simulink model "crossroad"  (R2023a)
settings: Solver=VariableStepDiscrete  StartTime=21600  StopTime=54000  FixedStep=1  MinStep=1  RelTol=1e-3
InitFcn:
  | clear S_code; % Resetta variabili persistent di una funzione
  | clear controllore_code;
  | clear controllore_code_NN;
  | clear sensor_S12 sensor_S3;
libraries: truetime x5, fuzblock x2
settings Model: SimulationMode=accelerator  NumberOfSteps=5  Creator=simmt  LastModifiedBy=simmt

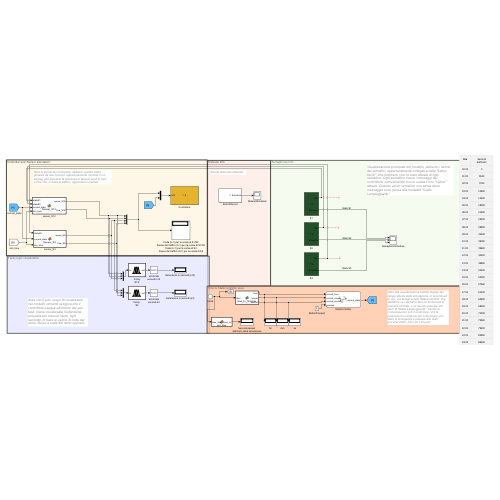
[thumbnail: Simulink's stored preview of the top-level diagram]
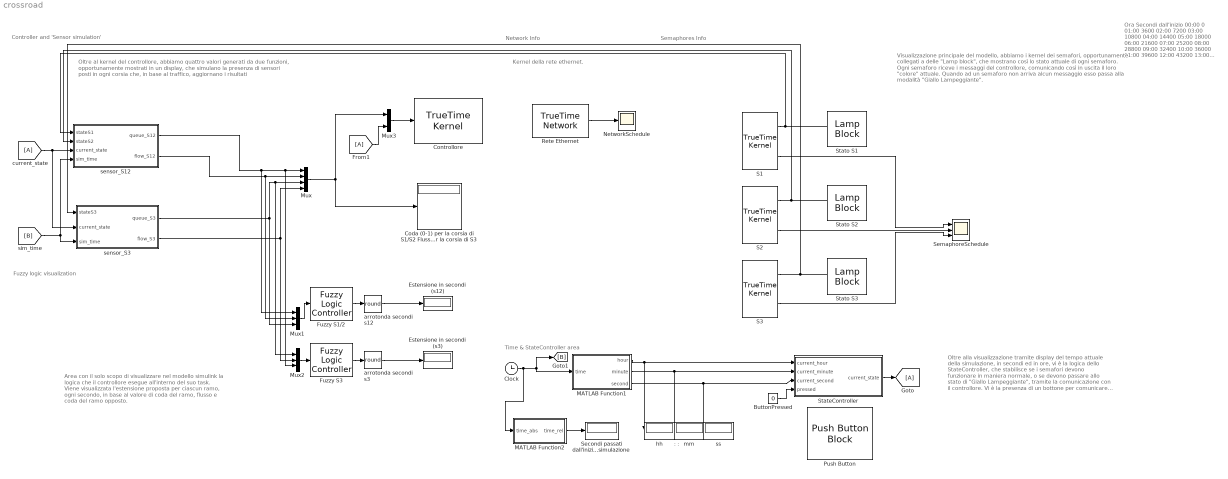
== system crossroad ==
  note: : :
  note: Ora
      | Secondi dall’inizio
      |
      | 00:00
      | 0
      |
      | 01:00
      | 3600
      |
      | 02:00
      | 7200
      |
      | 03:00
      | 10800
      |
      | 04:00
      | 14400
      |
      | 05:00
      | 18000
      |
      | 06:00
      | 21600
      |
      | 07:00
      | 25200
      |
      | 08:00
      | 28800
      |
      | 09:00
      | 32400
      |
      | 10:00
      | 36000
      |
      | 11:00
      | 39600
      |
      | 12:00
      | 43200
      |
      | 13:00
      | 46800
      |
      | 14:00
      | 50400
      |
      | 15:00
      | 54000
      |
      | 16:00
      | 57600
      |
      | 17:00
      | 61200
      |
      | 18:00
      | 64800
      |
      | 19:00
      | 68400
      |
      | 20:00
      | 72000
      |
      | 21:00
      | 75600
      |
      | 22:00
      | 79200
      |
      | 23:00
      | 82800
      |
      | 24:00
      | 86400
  note: Oltre al kernel del controllore, abbiamo quattro valori generati da due funzioni, opportunamente mostrati in un display, che simulano la presenza di sensori posti in ogni corsia che, in base al traffico, aggiornano i risultati
  note: Time & StateController area
  note: Controller and 'Sensor simulation'
  note: Semaphores Info
  note: Network Info
  note: Fuzzy logic visualization
  note: Area con il solo scopo di visualizzare nel modello simulink la logica che il controllore esegue all'interno del suo task. Viene visualizzata l'estensione proposta per ciascun ramo, ogni secondo, in base al valore di coda del ramo, flusso e coda del ramo opposto.
  note: Kernel della rete ethernet.
  note: Visualizzazione principale del modello, abbiamo i kernel dei semafori, opportunamente collegati a delle "Lamp block", che mostrano così lo stato attuale di ogni semaforo. Ogni semaforo riceve i messaggi del controllore, comunicando così in uscita il loro "colore" attuale. Quando ad un semaforo non arriva alcun messaggio esso passa alla modalità "Giallo Lampeggiante".
  note: Oltre alla visualizzazione tramite display del tempo attuale della simulazione, in secondi ed in ore, vi è la logica dello StateController, che stabilisce se i semafori devono funzionare in maniera normale, o se devono passare allo stato di "Giallo Lampeggiante", tramite la comunicazione con il controllore. Vi è la presenza di un bottone per comunicare uno stato di emergenza e passare allo stato poc'anzi citato. (clic con il mouse)
  "     mm     " : Display
  " ss" : Display
  ButtonPressed : Constant  Value=0  OutDataTypeStr=boolean
  Clock : Clock
  Coda (0-1) per la corsia di S1/S2 Flusso del traffico (0-1) per la corsia di S1/S2 Coda (0-1) per la corsia di S3 Flusso del traffico (0-1) per la corsia di S3 : Display
      settings: Format=bank
  Controllore : truetime/TrueTime Kernel  sfun=controllore_init  args=[]  ninputsoutputs=[5 0]  ntriggers=0  trigtype=falling  nwnodenbr=[1 4]  clockoffsetdrift=[0 0]  schedoutput=off  battery=off  poweroutput=off  label=1: 4
  Estensione in secondi (s12) : Display
      settings: Format=decimal (Stored Integer)
  Estensione in secondi (s3) : Display
  From1 : From
  Fuzzy S1/2 : fuzblock/Fuzzy Logic  Controller  FIS='green_extend.fis'  OutputSampleNumber=101  DataType=double  FuzzifiedInputs=off  RuleFiringStrengths=off  RuleOutputs=off  AggregatedOutputs=off  SimulateUsing=Interpreted execution  OutOfRangeInputValueMessage=warning  NoRuleFiredMessage=warning  EmptyOutputFuzzySetMessage=warning
  Fuzzy S3 : fuzblock/Fuzzy Logic  Controller  FIS='green_extend.fis'  OutputSampleNumber=101  DataType=double  FuzzifiedInputs=off  RuleFiringStrengths=off  RuleOutputs=off  AggregatedOutputs=off  SimulateUsing=Interpreted execution  OutOfRangeInputValueMessage=warning  NoRuleFiredMessage=warning  EmptyOutputFuzzySetMessage=warning
  Goto : Goto
  MATLAB Function1 : MATLAB Function  TreatAsAtomicUnit=on
  MATLAB Function2 : MATLAB Function  TreatAsAtomicUnit=on
  Mux : Mux
  Mux1 : Mux  Inputs=3
  Mux2 : Mux  Inputs=3
  Mux3 : Mux  Inputs=2
  NetworkSchedule : Scope
  Push Button : PushButtonBlock  ButtonText=Emergency  Icon=Hexagon  IconAlignment=Center  IconColor=On  OffValue=0.000000
  Rete Ethernet : truetime/TrueTime Network  nwtype=CSMA/CD (Ethernet)  nwnbr=1  nnodes=4  rate=20000000  minsize=512  lossprob=0.001  seed=42  bandwidths=[0.5 0.5]  slotsize=512  schedule=[1 1 2]  memsize=80000  buftype=Common buffer  overflow=Retransmit  dynSchedule=0  miniSlotSize=0  NIT=0  QSortMode=FIFO  sync=0  irtSchedule=0  nrtLength=0  nodeGraph=0  scheduleoutput=on
  S1 : truetime/TrueTime Kernel  sfun=S1_init  args=[]  ninputsoutputs=[0 1]  ntriggers=0  trigtype=falling  nwnodenbr=[1 1]  clockoffsetdrift=[0 0]  schedoutput=on  battery=off  poweroutput=off  label=1: 1
  S2 : truetime/TrueTime Kernel  sfun=S2_init  args=[]  ninputsoutputs=[0 1]  ntriggers=0  trigtype=falling  nwnodenbr=[1 2]  clockoffsetdrift=[0 0]  schedoutput=on  battery=off  poweroutput=off  label=1: 2
  S3 : truetime/TrueTime Kernel  sfun=S3_init  args=[]  ninputsoutputs=[0 1]  ntriggers=0  trigtype=falling  nwnodenbr=[1 3]  clockoffsetdrift=[0 0]  schedoutput=on  battery=off  poweroutput=off  label=1: 3
  Secondi passati dall'inizio della simulazione : Display
  SemaphoreSchedule : Scope  NumInputPorts=3
  StateController : Stateflow chart  TreatAsAtomicUnit=on
  Stato S1 : LampBlock  LabelPosition=Hide
  Stato S2 : LampBlock  LabelPosition=Hide
  Stato S3 : LampBlock  LabelPosition=Hide
  arrotonda secondi s12 : Rounding  Operator=round
  arrotonda secondi s3 : Rounding  Operator=round
  current_state : From
  hh : Display
  sensor_S12 : MATLAB Function  TreatAsAtomicUnit=on  SystemSampleTime=1
  sensor_S3 : MATLAB Function  TreatAsAtomicUnit=on  SystemSampleTime=1
  wires:
  sensor_S12/1(queue_S12) -> Mux1/1, Mux2/3, Mux/1
  Rete Ethernet/1 -> NetworkSchedule/1
  S3/2 -> SemaphoreSchedule/3
  S1/1 -> sensor_S12/1(stateS1)
  S2/1 -> sensor_S12/2(stateS2)
  S3/1 -> sensor_S3/1(stateS3)
  Mux/1 -> Coda (0-1) per la corsia di S1/S2 Flusso del traffico (0-1) per la corsia di S1/S2 Coda (0-1) per la corsia di S3 Flusso del traffico (0-1) per la corsia di S3/1, Mux3/1
  Clock/1 -> [B], MATLAB Function1/1(time), MATLAB Function2/1(time_abs)
  MATLAB Function1/1(hour) -> hh/1, StateController/1(current_hour)
  StateController/1(current_state) -> Goto/1
  S1/2 -> SemaphoreSchedule/1
  S2/2 -> SemaphoreSchedule/2
  ButtonPressed/1 -> StateController/4(pressed)
  From1/1 -> Mux3/2
  Mux3/1 -> Controllore/1
  sensor_S3/1(queue_S3) -> Mux2/1, Mux/3, Mux1/3
  sensor_S12/2(flow_S12) -> Mux1/2, Mux/2
  sensor_S3/2(flow_S3) -> Mux/4, Mux2/2
  Mux1/1 -> Fuzzy S1/2/1
  Mux2/1 -> Fuzzy S3/1
  Fuzzy S3/1 -> arrotonda secondi s3/1
  Fuzzy S1/2/1 -> arrotonda secondi s12/1
  arrotonda secondi s12/1 -> Estensione in secondi (s12)/1
  arrotonda secondi s3/1 -> Estensione in secondi (s3)/1
  MATLAB Function1/2(minute) -> "     mm     "/1, StateController/2(current_minute)
  current_state/1 -> sensor_S3/2(current_state), sensor_S12/3(current_state)
  [B] -> sensor_S12/4(sim_time), sensor_S3/3(sim_time)
  MATLAB Function1/3(second) -> " ss"/1, StateController/3(current_second)
  MATLAB Function2/1(time_rel) -> Secondi passati dall'inizio della simulazione/1

== matlab function crossroad/MATLAB Function1 ==
  data: time input; hour output; minute output; second output
function [hour, minute, second] = time_to_hhmmss(time)
% time in hh:mm:ss

t = mod(time, 24*3600);

hour   = floor(t/3600);          % 0..23
minute = floor(mod(t,3600)/60);  % 0..59
second = floor(mod(t,60));       % 0..59
end

== matlab function crossroad/MATLAB Function2 ==
  data: time_abs input; time_rel output
function time_rel = sim_time(time_abs)
% time_abs  : tempo assoluto di simulazione (da clock), in secondi
% time_rel  : secondi trascorsi dall'inizio simulazione (1,2,3,...)

persistent tStart
if isempty(tStart)
    tStart = time_abs;   % istante di start (es. 43200)
end

elapsed = time_abs - tStart;    % può avere decimali
elapsed = floor(elapsed);       % 0,1,2,... interi
time_rel = elapsed + 1;        % parte da 1 invece che da 0

== stateflow chart crossroad/StateController ==
  state EmergencyCall
    entry:
    EmergencyFlag = 1;
    fprintf('[%02.0f:%02.0f:%02.0f][StateController]: Rilevato bottone di emergenza, stato di emergenza chiamato.\n', ...
    current_hour, current_minute, current_second);
  state FlashingYellow
    entry:
    current_state = 2;
    if EmergencyFlag == 0
    fprintf('[%02.0f:%02.0f:%02.0f][StateController]: Modalità Giallo Lampeggiante notturna.\n', ...
    current_hour, current_minute, current_second);
    elseif EmergencyFlag == 1
    fprintf(['[%02.0f:%02.0f:%02.0f][StateController]: Modalità Giallo Lampeggiante, ' ...
    'emergenza in corso.\n'], ...
    current_hour, current_minute, current_second);
    end
  state NormalState
    entry:
    fprintf('[%02.0f:%02.0f:%02.0f][StateController]: Modalità Normale.\n', ...
    current_hour, current_minute, current_second);
    current_state = 1;
  state EmergencyCall1
    entry:
    fprintf('[%02.0f:%02.0f:%02.0f][StateController]: Rilevato bottone di emergenza.\n', ...
    current_hour, current_minute, current_second);
    if EmergencyFlag == 0
    EmergencyFlag = 1;
    fprintf('[%02.0f:%02.0f:%02.0f][StateController]: Stato di emergenza chiamato.\n', ...
    current_hour, current_minute, current_second);
    elseif EmergencyFlag == 1
    EmergencyFlag = 0;
    fprintf('[%02.0f:%02.0f:%02.0f][StateController]: Emergenza finita.\n', ...
    current_hour, current_minute, current_second);
    end
  NormalState -> EmergencyCall [order 2] : [pressed == 1 && after(0.2,sec)]
  EmergencyCall -> FlashingYellow : [after(0.2, sec)]
  (default) -> NormalState
  FlashingYellow -> NormalState [order 1] : [current_hour >= 6 && current_hour <= 22 && EmergencyFlag ~= 1]
  NormalState -> FlashingYellow [order 1] : [current_hour >= 22]
  EmergencyCall1 -> NormalState [order 2] : [current_hour >= 6 && current_hour <= 22 && after(0.2, sec)]
  FlashingYellow -> EmergencyCall1 [order 2] : [pressed == 1 && after(0.2,sec)]
  EmergencyCall1 -> FlashingYellow [order 1] : [(current_hour >= 22 || current_hour < 6) && after(0.2, sec)]
  data: current_hour input; current_state output; EmergencyFlag local double =0; current_minute input; current_second input; pressed input boolean

== matlab function crossroad/sensor_S12 ==
  data: stateS1 input; queue_S12 output; stateS2 input; flow_S12 output; current_state input; sim_time input
function [queue_S12, flow_S12] = Sensor_S12(stateS1, stateS2, current_state, sim_time)
% Sensor_S12 - Sensore aggregato per il ramo S1/S2 (4 corsie)
% stateS1, stateS2: 1=rosso, 2=giallo, 3=verde
% current_state: 1 = normale, 2 = giallo lampeggiante
% queue_S12: coda normalizzata [0,1]
% flow_S12 : flusso medio normalizzato [0,1]
% sim_time: normalizza l'uscita del Clock


% Parametri
% ==========================================================
SEED_S12 = uint32(5);    % per simulazioni diverse

queue_max = 60;    % coda piena = 60 veicoli (4 corsie)
C_max     = 3;     % max veicoli che possono uscire in 1 s (verde)
flow_max  = 2.5;     % flusso medio massimo atteso (veicoli/s)
Nwin      = 5;     % finestra per media flusso (5 s)
% ==========================================================


% Stato interno tra un passo e l'altro
persistent queue arrivalsWindow
if isempty(queue)
    queue = 25;                      % coda iniziale
end
if isempty(arrivalsWindow)
    arrivalsWindow = zeros(Nwin,1); % finestra iniziale di zeri
end


% RNG locale con seed (codegen-friendly)
% ==========================================================
persistent rngState seedUsed lastSimTime

% Inizializza SEMPRE le persistent prima di qualunque uso
if isempty(rngState)
    rngState = uint32(1);
end
if isempty(seedUsed)
    seedUsed = uint32(0);
end
if isempty(lastSimTime)
    lastSimTime = -inf;
end

newRun = (sim_time < lastSimTime);
lastSimTime = sim_time;

if newRun || (seedUsed ~= SEED_S12)
    rngState = SEED_S12;
    if rngState == 0
        rngState = uint32(1);
    end
    seedUsed = SEED_S12;
end
% ==========================================================


% profilo orario
hour_of_day   = floor(mod(sim_time/3600, 24));      % 0..23
minute_of_day = floor(mod(sim_time,3600)/60);       % 0..59
second_of_day = floor(mod(sim_time,60));            % 0..59


% Genera arrivi casuali per corsia (4 corsie)
% ==========================================================
if (hour_of_day >= 7 && hour_of_day < 9)
    p_arr_S12 = 0.30;
elseif (hour_of_day >= 9 && hour_of_day < 12)
    p_arr_S12 = 0.26;
elseif (hour_of_day >= 12 && hour_of_day < 14)
    p_arr_S12 = 0.33;
elseif (hour_of_day >= 18 && hour_of_day < 20)
    p_arr_S12 = 0.30;
elseif (hour_of_day >= 22 || hour_of_day < 6)
    p_arr_S12 = 0.02;
else
    p_arr_S12 = 0.22;
end

% arrivi = sum(rand(4,1) < p_arr_S12); % (linea senza uso di SEED) @@@
arrivi = 0;
for k = 1:4
    [rngState, r] = randu_xorshift32(rngState);
    if r < p_arr_S12
        arrivi = arrivi + 1;
    end
end
% ==========================================================

% Verifica se S1/S2 hanno il verde
hasGreen = (stateS1 == 3) || (stateS2 == 3);

% Timer verde — conta i secondi consecutivi di verde
persistent greenTimer
if isempty(greenTimer), greenTimer = 0; end

% Calcola quante auto escono
% ==========================================================
if hasGreen
    greenTimer = greenTimer + 1;
else
    greenTimer = 0;
end

if current_state == 1
    if hasGreen
        uscita_teorica = min(C_max, queue);
        [rngState, r] = randu_xorshift32(rngState);
        if greenTimer > 20
            fattore = 0.75 + 0.25*r;  % 0.75–1.00, media 0.875
        else
            fattore = 0.55 + 0.45*r;  % 0.55–1.00, media 0.775
        end

        uscita = min(queue, round(fattore * uscita_teorica));
    else
        uscita = 0;
    end

elseif current_state == 2
    uscita_teorica = min(C_max, queue);
    % fattore = 0.3 + 0.4*rand();               % (linea senza uso di SEED) @@@
    [rngState, r] = randu_xorshift32(rngState);
    fattore = 0.3 + 0.4*r;                      % 30–70% del max
    uscita  = min(queue, round(fattore * uscita_teorica));
else
    uscita = 0;
end
% ==========================================================


% Aggiorna coda
queue = queue + arrivi - uscita;
if queue < 0, queue = 0; end
if queue > 80, queue = 80; end

% Aggiorna finestra arrivi per stima flusso medio
arrivalsWindow = [arrivalsWindow(2:end); arrivi];
flowMedia = mean(arrivalsWindow);   % veicoli/s medi sugli ultimi Nwin secondi


% Normalizza per dare in uscita [0,1]
% ==========================================================
queue_S12 = queue / queue_max;
if queue_S12 > 1
    queue_S12 = 1;
end

%----------------@DEBUG@----------------
%fprintf('[%02.0f:%02.0f:%02.0f][sensor_S12]: S1  queue = %.0f veicoli (norm = %.2f)\n', ...
%    hour_of_day, minute_of_day, second_of_day, queue, queue_S12);
%--------------------------------------

flow_S12 = flowMedia / flow_max;
if flow_S12 > 1
    flow_S12 = 1;
end
% ==========================================================

end


function [state, u] = randu_xorshift32(state)
% RNG uniforme [0,1) con stato uint32 (xorshift32)
state = bitxor(state, bitshift(state, 13));
state = bitxor(state, bitshift(state, -17));
state = bitxor(state, bitshift(state, 5));
u = double(state) * 2.3283064365386963e-10; % 1/2^32
end

== matlab function crossroad/sensor_S3 ==
  data: stateS3 input; queue_S3 output; flow_S3 output; current_state input; sim_time input
function [queue_S3, flow_S3] = Sensor_S3(stateS3, current_state, sim_time)
% Sensor_S3 - Sensore aggregato per il ramo S3 (2 corsie)
% stateS3: 1=rosso, 2=giallo, 3=verde
% current_state: 1 = normale, 2 = giallo lampeggiante
% queue_S3: coda normalizzata [0,1]
% flow_S3 : flusso medio normalizzato [0,1]
% sim_time: tempo simulazione in secondi (uscita del Clock)


% Parametri
% ==========================================================
SEED_S3 = uint32(6);    % simulazioni diverse

queue_max = 40;    % coda piena = 40 veicoli (2 corsie)
C_max     = 2;     % max veicoli che possono uscire in 1 s (verde)
flow_max  = 1.2;   % flusso max realistico (2 corsie, picco ~1.1 veic/s)
Nwin      = 5;     % finestra per media flusso (5 s)
% ==========================================================


% Stato interno tra un passo e l'altro
persistent queue arrivalsWindow
if isempty(queue)
    queue = 10;
end
if isempty(arrivalsWindow)
    arrivalsWindow = zeros(Nwin,1);
end

% RNG locale con seed (codegen-friendly)
% ==========================================================
persistent rngState seedUsed lastSimTime

% Inizializza SEMPRE le persistent prima di qualunque uso
if isempty(rngState)
    rngState = uint32(1);
end
if isempty(seedUsed)
    seedUsed = uint32(0);
end
if isempty(lastSimTime)
    lastSimTime = -inf;
end

newRun = (sim_time < lastSimTime);
lastSimTime = sim_time;

if newRun || (seedUsed ~= SEED_S3)
    rngState = SEED_S3;
    if rngState == 0
        rngState = uint32(1);   % evita stato nullo
    end
    seedUsed = SEED_S3;
end
% ==========================================================


% --- profilo orario ---
hour_of_day   = floor(mod(sim_time/3600, 24));      % 0..23
minute_of_day = floor(mod(sim_time,3600)/60);       % 0..59
second_of_day = floor(mod(sim_time,60));            % 0..59 %#ok<NASGU>


% Genera arrivi casuali per corsia (2 corsie)
% S3 ramo secondario
% ==========================================================
if (hour_of_day >= 7 && hour_of_day < 9)
    p_arr_S3 = 0.32;
elseif (hour_of_day >= 9 && hour_of_day < 12)
    p_arr_S3 = 0.28;
elseif (hour_of_day >= 12 && hour_of_day < 14)
    p_arr_S3 = 0.35;
elseif (hour_of_day >= 18 && hour_of_day < 20)
    p_arr_S3 = 0.32;
elseif (hour_of_day >= 22 || hour_of_day < 6)
    p_arr_S3 = 0.02;
else
    p_arr_S3 = 0.24;
end


% arrivi = sum(rand(2,1) < p_arr_S3); % (linea senza uso di SEED) @@@
arrivi = 0;
for k = 1:2
    [rngState, r] = randu_xorshift32(rngState);
    if r < p_arr_S3
        arrivi = arrivi + 1;
    end
end
% ==========================================================

% Semaforo verde?
hasGreen = (stateS3 == 3);

% Timer verde — conta i secondi consecutivi di verde
persistent greenTimer
if isempty(greenTimer), greenTimer = 0; end

% Calcola quante auto escono
% ==========================================================
if hasGreen
    greenTimer = greenTimer + 1;
else
    greenTimer = 0;
end

if current_state == 1
    if hasGreen
        uscita_teorica = min(C_max, queue);
        [rngState, r] = randu_xorshift32(rngState);
        if greenTimer > 20
            fattore = 0.70 + 0.30*r;  % 0.70–1.00, media 0.850
        else
            fattore = 0.50 + 0.50*r;  % 0.50–1.00, media 0.750
        end


        uscita = min(queue, round(fattore * uscita_teorica));
    else
        uscita = 0;
    end

elseif current_state == 2
    uscita_teorica = min(C_max, queue);         % stesso limite massimo
    % fattore = 0.3 + 0.4*rand();               % (linea senza uso di SEED) @@@
    [rngState, r] = randu_xorshift32(rngState);
    fattore = 0.3 + 0.4*r;                      % 30–70% del max
    uscita  = min(queue, round(fattore * uscita_teorica));
else
    uscita = 0;
end
% ==========================================================


% Aggiorna coda
queue = queue + arrivi - uscita;
if queue < 0, queue = 0; end
if queue > 60, queue = 60; end


% Aggiorna finestra arrivi per stima flusso
arrivalsWindow = [arrivalsWindow(2:end); arrivi];
flowMedia = mean(arrivalsWindow);


% Normalizza
% ==========================================================
queue_S3 = queue / queue_max;
if queue_S3 > 1
    queue_S3 = 1;
end

%----------------@DEBUG@----------------
%fprintf('[%02.0f:%02.0f:%02.0f][sensor_S3]: S3  queue = %.0f veicoli (norm = %.2f)\n', ...
%    hour_of_day, minute_of_day, second_of_day, queue, queue_S3);
%--------------------------------------

flow_S3 = flowMedia / flow_max;
if flow_S3 > 1
    flow_S3 = 1;
end
% ==========================================================

end


function [state, u] = randu_xorshift32(state)
% RNG uniforme [0,1) con stato uint32 (xorshift32)
state = bitxor(state, bitshift(state, 13));
state = bitxor(state, bitshift(state, -17));
state = bitxor(state, bitshift(state, 5));
u = double(state) * 2.3283064365386963e-10; % 1/2^32
end
